simulink model "pot_field_1obs"  (R2016a)
settings: Solver=VariableStepAuto  StartTime=0.0  StopTime=inf  RelTol=1e-3
undefined symbols (not defined in the file): Speed, Yaw
libraries: robotlib x3
settings Model: Creator=nmanzini  LastModifiedBy=nmanzini

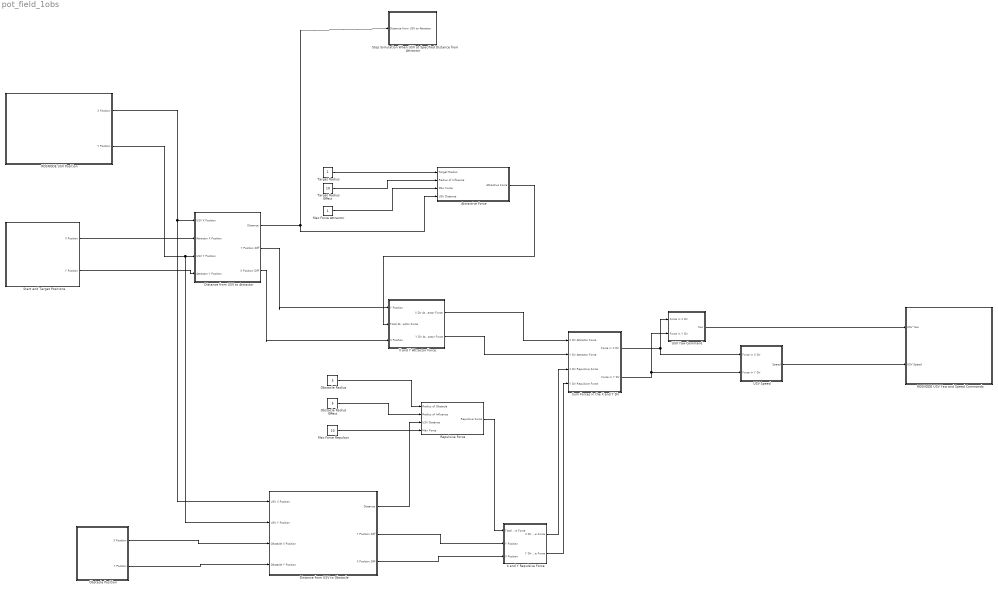
== system pot_field_1obs ==
  Attractive Force : Subsystem
  Distance from USV to Attractor : Subsystem
  Distance from USV to Obstacle : Subsystem
  Max Force Attractor : Constant  OutDataTypeStr=Inherit: Inherit via back propagation
  Max Force Repulsor : Constant  Value=10  OutDataTypeStr=Inherit: Inherit via back propagation
  "Obstacle Position " : Subsystem
  Obstacle Radius : Constant  Value=5  OutDataTypeStr=Inherit: Inherit via back propagation
  Obstacle Radius Effect : Constant  Value=5  OutDataTypeStr=Inherit: Inherit via back propagation
  ROSNODE USV Position : Subsystem
  ROSNODE USV Yaw and Speed Commands : Subsystem
  Repulsive Force : Subsystem
  Start and Target Positions : Subsystem
  Stop Simulation When USV at Specified Distance from Attractor : Subsystem
  Sum Forces in the X and Y Dir : Subsystem
  Target Radius : Constant  OutDataTypeStr=Inherit: Inherit via back propagation
  Target Radius Effect : Constant  Value=10  OutDataTypeStr=Inherit: Inherit via back propagation
  USV Speed : Subsystem
  USV Yaw Command : Subsystem
  X and Y Attractor Force : Subsystem
  X and Y Repulsive Force : Subsystem
  wires:
  Obstacle Radius/1 -> Repulsive Force/1("Radius of Obstacle ")
  Obstacle Radius Effect/1 -> Repulsive Force/2(Radius of Influence)
  Max Force Repulsor/1 -> Repulsive Force/4(Max Force)
  Repulsive Force/1(Repulsive Force) -> X and Y Repulsive Force/1(Total Repulsive Force)
  Distance from USV to Attractor/1(Distance) -> Attractive Force/4(USV Distance), Stop Simulation When USV at Specified Distance from Attractor/1(Distance from USV to Attractor)
  Start and Target Positions/1(X Position) -> Distance from USV to Attractor/2(Attractor X Position)
  Start and Target Positions/2(Y Position) -> Distance from USV to Attractor/4(Attractor Y Position)
  Distance from USV to Attractor/2(Y Position Diff) -> X and Y Attractor Force/1(Y Position)
  Distance from USV to Attractor/3(X Position Diff) -> X and Y Attractor Force/3("X Position ")
  Target Radius/1 -> Attractive Force/1(Target Radius)
  Target Radius Effect/1 -> Attractive Force/2(Radius of Influence)
  Max Force Attractor/1 -> Attractive Force/3(Max Force)
  Attractive Force/1(Attractive Force) -> X and Y Attractor Force/2(Total Attractor Force)
  Sum Forces in the X and Y Dir/1(Force in X Dir) -> USV Yaw Command/1(Force in X Dir), USV Speed/1(Force in X Dir)
  Sum Forces in the X and Y Dir/2(Force in Y Dir) -> USV Yaw Command/2("Force in Y Dir "), USV Speed/2(Force in Y Dir)
  X and Y Attractor Force/1(X Dir Attractor Force) -> Sum Forces in the X and Y Dir/1(X Dir Attractor Force)
  X and Y Attractor Force/2(Y Dir Attractor Force) -> Sum Forces in the X and Y Dir/2(Y Dir Attractor Force)
  X and Y Repulsive Force/1(X Dir Repulsive Force) -> Sum Forces in the X and Y Dir/3(X Dir Repulsive Force)
  X and Y Repulsive Force/2(Y Dir Repulsive Force) -> Sum Forces in the X and Y Dir/4("Y Dir Repulsive Force ")
  USV Yaw Command/1(Yaw) -> ROSNODE USV Yaw and Speed Commands/1(USV Yaw)
  USV Speed/1(Speed) -> ROSNODE USV Yaw and Speed Commands/2(USV Speed)
  ROSNODE USV Position/1(X Position) -> Distance from USV to Obstacle/1("USV X Position "), Distance from USV to Attractor/1(USV X Position)
  ROSNODE USV Position/2(Y Position) -> Distance from USV to Obstacle/2(USV Y Position), Distance from USV to Attractor/3(USV Y Position)
  Distance from USV to Obstacle/1(Distance) -> Repulsive Force/3(USV Distance)
  Distance from USV to Obstacle/2(Y Position Diff) -> X and Y Repulsive Force/2(Y Position)
  Distance from USV to Obstacle/3(X Position Diff) -> X and Y Repulsive Force/3(X Position)
  "Obstacle Position "/1(X Position) -> Distance from USV to Obstacle/3(Obstacle X Position)
  "Obstacle Position "/2(Y Position) -> Distance from USV to Obstacle/4(Obstacle Y Position)

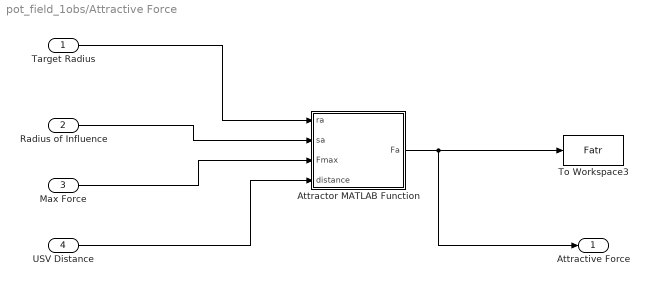
== system pot_field_1obs/Attractive Force ==
  Target Radius : Inport
  Radius of Influence : Inport  Port=2
  Max Force : Inport  Port=3
  USV Distance : Inport  Port=4
  Attractor MATLAB Function : MATLAB Function  TreatAsAtomicUnit=on
  To Workspace3 : ToWorkspace  VariableName=Fatr  SaveFormat=Timeseries  SampleTime=-1
  Attractive Force : Outport
  wires:
  Max Force/1 -> Attractor MATLAB Function/3(Fmax)
  USV Distance/1 -> Attractor MATLAB Function/4(distance)
  Attractor MATLAB Function/1(Fa) -> Attractive Force/1, To Workspace3/1
  Target Radius/1 -> Attractor MATLAB Function/1(ra)
  Radius of Influence/1 -> Attractor MATLAB Function/2(sa)

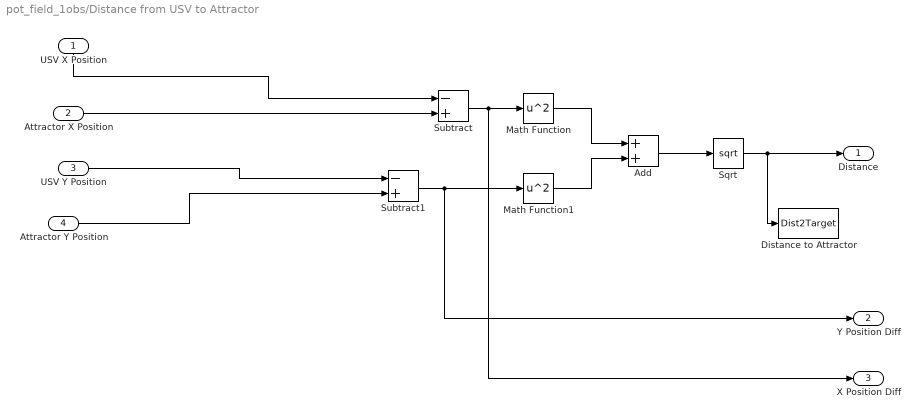
== system pot_field_1obs/Distance from USV to Attractor ==
  USV X Position : Inport
  Attractor X Position : Inport  Port=2
  USV Y Position : Inport  Port=3
  Attractor Y Position : Inport  Port=4
  Add : Sum  OutDataTypeStr=Inherit: Inherit via back propagation
  Distance to Attractor : ToWorkspace  VariableName=Dist2Target  SaveFormat=Timeseries  SampleTime=-1
  Math Function : Math  Operator=square  OutDataTypeStr=Inherit: Inherit via back propagation  SaturateOnIntegerOverflow=on
  Math Function1 : Math  Operator=square  OutDataTypeStr=Inherit: Inherit via back propagation  SaturateOnIntegerOverflow=on
  Sqrt : Sqrt  OutDataTypeStr=Inherit: Inherit via back propagation  SaturateOnIntegerOverflow=on
  Subtract : Sum  Inputs=-+  OutDataTypeStr=Inherit: Inherit via back propagation
  Subtract1 : Sum  Inputs=-+  OutDataTypeStr=Inherit: Inherit via back propagation
  Distance : Outport
  Y Position Diff : Outport  Port=2
  X Position Diff : Outport  Port=3
  wires:
  Attractor Y Position/1 -> Subtract1/2
  USV Y Position/1 -> Subtract1/1
  USV X Position/1 -> Subtract/1
  Attractor X Position/1 -> Subtract/2
  Subtract1/1 -> Y Position Diff/1, Math Function1/1
  Subtract/1 -> X Position Diff/1, Math Function/1
  Math Function/1 -> Add/1
  Math Function1/1 -> Add/2
  Add/1 -> Sqrt/1
  Sqrt/1 -> Distance/1, Distance to Attractor/1

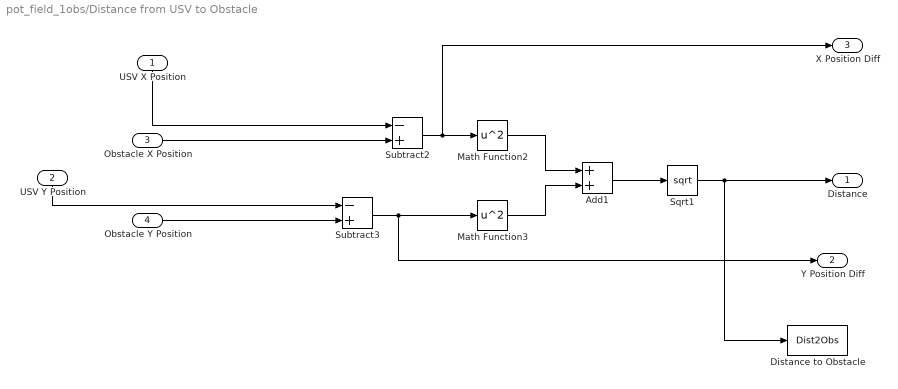
== system pot_field_1obs/Distance from USV to Obstacle ==
  "USV X Position " : Inport
  USV Y Position : Inport  Port=2
  Obstacle X Position : Inport  Port=3
  Obstacle Y Position : Inport  Port=4
  Add1 : Sum  OutDataTypeStr=Inherit: Inherit via back propagation
  Distance to Obstacle : ToWorkspace  VariableName=Dist2Obs  SaveFormat=Timeseries  SampleTime=-1
  Math Function2 : Math  Operator=square  OutDataTypeStr=Inherit: Inherit via back propagation  SaturateOnIntegerOverflow=on
  Math Function3 : Math  Operator=square  OutDataTypeStr=Inherit: Inherit via back propagation  SaturateOnIntegerOverflow=on
  Sqrt1 : Sqrt  OutDataTypeStr=Inherit: Inherit via back propagation  SaturateOnIntegerOverflow=on
  Subtract2 : Sum  Inputs=-+  OutDataTypeStr=Inherit: Inherit via back propagation
  Subtract3 : Sum  Inputs=-+  OutDataTypeStr=Inherit: Inherit via back propagation
  Distance : Outport
  Y Position Diff : Outport  Port=2
  X Position Diff : Outport  Port=3
  wires:
  Sqrt1/1 -> Distance/1, Distance to Obstacle/1
  Subtract3/1 -> Y Position Diff/1, Math Function3/1
  Subtract2/1 -> X Position Diff/1, Math Function2/1
  Obstacle X Position/1 -> Subtract2/2
  "USV X Position "/1 -> Subtract2/1
  Obstacle Y Position/1 -> Subtract3/2
  USV Y Position/1 -> Subtract3/1
  Math Function2/1 -> Add1/1
  Math Function3/1 -> Add1/2
  Add1/1 -> Sqrt1/1

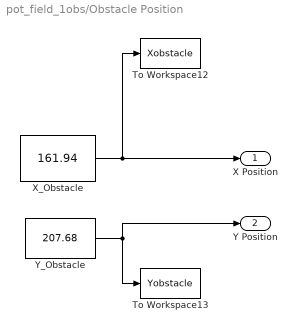
== system pot_field_1obs/Obstacle Position  ==
  To Workspace12 : ToWorkspace  VariableName=Xobstacle  SaveFormat=Timeseries  SampleTime=-1
  To Workspace13 : ToWorkspace  VariableName=Yobstacle  SaveFormat=Timeseries  SampleTime=-1
  "X_Obstacle " : Constant  Value=161.94  OutDataTypeStr=Inherit: Inherit via back propagation
  Y_Obstacle : Constant  Value=207.68  OutDataTypeStr=Inherit: Inherit via back propagation
  X Position : Outport
  Y Position : Outport  Port=2
  wires:
  "X_Obstacle "/1 -> X Position/1, To Workspace12/1
  Y_Obstacle/1 -> Y Position/1, To Workspace13/1

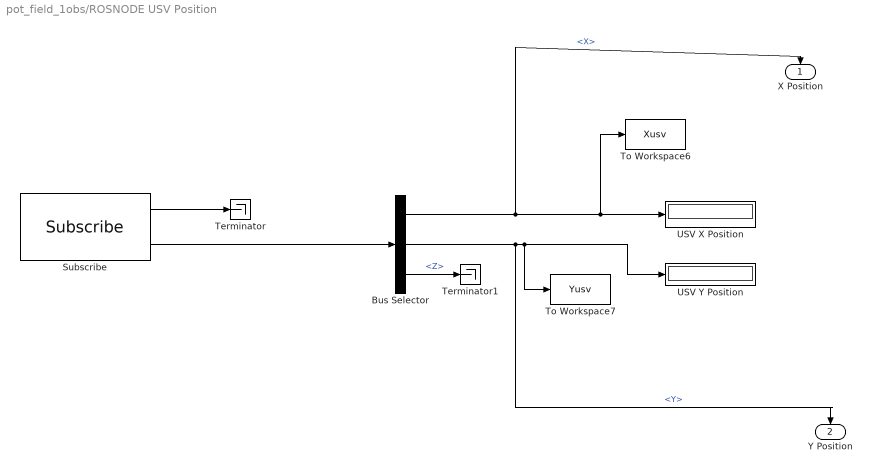
== system pot_field_1obs/ROSNODE USV Position ==
  Bus Selector : BusSelector  OutputSignals=Pose.Pose.Position.X,Pose.Pose.Position.Y,Pose.Pose.Position.Z
  Subscribe : robotlib/Subscribe  SourceLibraryInfo=This block requires Robotics System Toolbox  topicSource=Select from ROS network  topic=/geonav_odom  messageType=nav_msgs/Odometry  sampleTime=-1  messageQueueLength=1000
  Terminator : Terminator
  Terminator1 : Terminator
  To Workspace6 : ToWorkspace  VariableName=Xusv  SaveFormat=Timeseries  SampleTime=-1
  To Workspace7 : ToWorkspace  VariableName=Yusv  SaveFormat=Timeseries  SampleTime=-1
  USV X Position : Display
  USV Y Position : Display
  X Position : Outport
  Y Position : Outport  Port=2
  wires:
  Subscribe/1 -> Terminator/1
  Bus Selector/3 -> Terminator1/1  "<Z>"
  Bus Selector/1 -> X Position/1, To Workspace6/1, USV X Position/1  "<X>"
  Subscribe/2 -> Bus Selector/1
  Bus Selector/2 -> USV Y Position/1, To Workspace7/1, Y Position/1  "<Y>"

== system pot_field_1obs/ROSNODE USV Yaw and Speed Commands ==
  USV Yaw : Inport
  USV Speed : Inport  Port=2
  Blank Message : robotlib/Blank Message  SourceLibraryInfo=This block requires Robotics System Toolbox  messageType=kingfisher_msgs/Course  SampleTime=inf
  Bus Assignment : BusAssignment  AssignedSignals=Yaw,Speed
  Publish1 : robotlib/Publish  SourceLibraryInfo=This block requires Robotics System Toolbox  topicSource=Select from ROS network  topic=/cmd_course  messageType=kingfisher_msgs/Course  messageQueueLength=1
  wires:
  USV Speed/1 -> Bus Assignment/3
  USV Yaw/1 -> Bus Assignment/2
  Blank Message/1 -> Bus Assignment/1
  Bus Assignment/1 -> Publish1/1

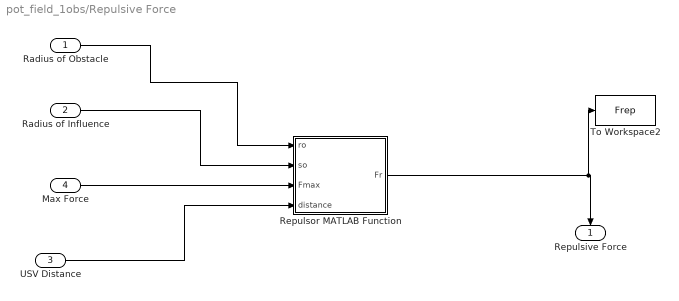
== system pot_field_1obs/Repulsive Force ==
  "Radius of Obstacle " : Inport
  Radius of Influence : Inport  Port=2
  USV Distance : Inport  Port=3
  Max Force : Inport  Port=4
  Repulsor MATLAB Function : MATLAB Function  TreatAsAtomicUnit=on
  To Workspace2 : ToWorkspace  VariableName=Frep  SaveFormat=Timeseries  SampleTime=-1
  Repulsive Force : Outport
  wires:
  USV Distance/1 -> Repulsor MATLAB Function/4(distance)
  Repulsor MATLAB Function/1(Fr) -> Repulsive Force/1, To Workspace2/1
  Max Force/1 -> Repulsor MATLAB Function/3(Fmax)
  Radius of Influence/1 -> Repulsor MATLAB Function/2(so)
  "Radius of Obstacle "/1 -> Repulsor MATLAB Function/1(ro)

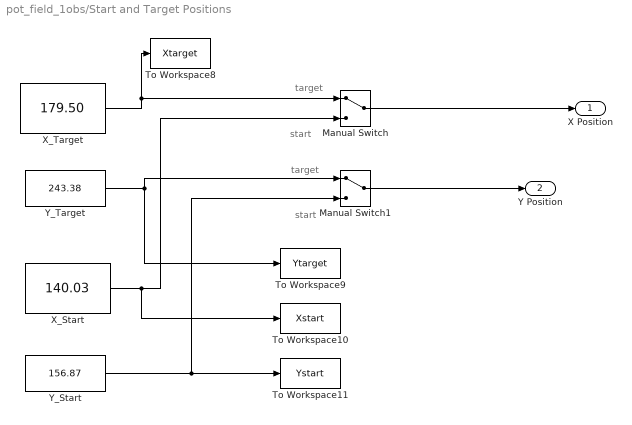
== system pot_field_1obs/Start and Target Positions ==
  note: target
  note: target
  note: start
  note: start
  Manual Switch : ManualSwitch
  Manual Switch1 : ManualSwitch
  To Workspace10 : ToWorkspace  VariableName=Xstart  SaveFormat=Timeseries  SampleTime=-1
  To Workspace11 : ToWorkspace  VariableName=Ystart  SaveFormat=Timeseries  SampleTime=-1
  To Workspace8 : ToWorkspace  VariableName=Xtarget  SaveFormat=Timeseries  SampleTime=-1
  To Workspace9 : ToWorkspace  VariableName=Ytarget  SaveFormat=Timeseries  SampleTime=-1
  X_Start : Constant  Value=140.03  OutDataTypeStr=Inherit: Inherit via back propagation
  X_Target : Constant  Value=179.50  OutDataTypeStr=Inherit: Inherit via back propagation
  Y_Start : Constant  Value=156.87  OutDataTypeStr=Inherit: Inherit via back propagation
  Y_Target : Constant  Value=243.38  OutDataTypeStr=Inherit: Inherit via back propagation
  X Position : Outport
  Y Position : Outport  Port=2
  wires:
  X_Target/1 -> To Workspace8/1, Manual Switch/1
  Manual Switch/1 -> X Position/1
  X_Start/1 -> To Workspace10/1, Manual Switch/2
  Y_Target/1 -> To Workspace9/1, Manual Switch1/1
  Manual Switch1/1 -> Y Position/1
  Y_Start/1 -> To Workspace11/1, Manual Switch1/2

== system pot_field_1obs/Stop Simulation When USV at Specified Distance from Attractor ==
  Distance from USV to Attractor : Inport
  Display1 : Display
  Stop Gain1 : Constant  Value=0  OutDataTypeStr=Inherit: Inherit via back propagation
  Stop Gain2 : Constant  OutDataTypeStr=Inherit: Inherit via back propagation
  Stop Simulation : Stop
  Stop Simulation Switch at distance from Target : Switch  Criteria=u2 > Threshold  Threshold=1.5
  wires:
  Distance from USV to Attractor/1 -> Stop Simulation Switch at distance from Target/2
  Stop Simulation Switch at distance from Target/1 -> Display1/1, Stop Simulation/1
  Stop Gain1/1 -> Stop Simulation Switch at distance from Target/1
  Stop Gain2/1 -> Stop Simulation Switch at distance from Target/3

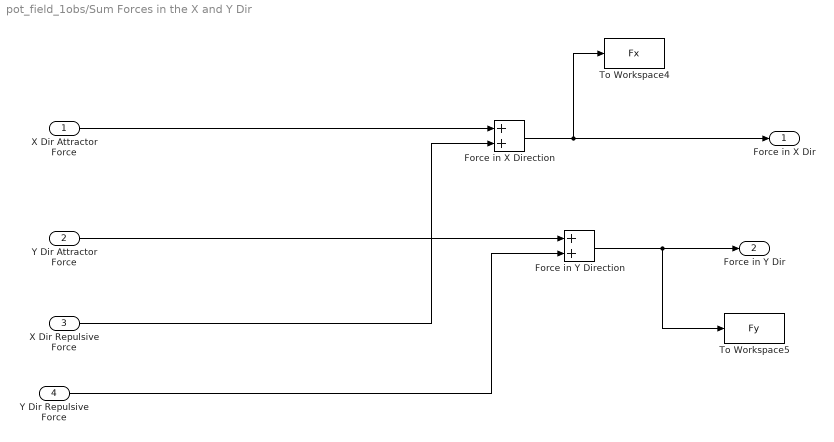
== system pot_field_1obs/Sum Forces in the X and Y Dir ==
  X Dir Attractor Force : Inport
  Y Dir Attractor Force : Inport  Port=2
  X Dir Repulsive Force : Inport  Port=3
  "Y Dir Repulsive Force " : Inport  Port=4
  Force in X Direction : Sum  OutDataTypeStr=Inherit: Inherit via back propagation
  Force in Y Direction : Sum  OutDataTypeStr=Inherit: Inherit via back propagation
  To Workspace4 : ToWorkspace  VariableName=Fx  SaveFormat=Timeseries  SampleTime=-1
  To Workspace5 : ToWorkspace  VariableName=Fy  SaveFormat=Timeseries  SampleTime=-1
  Force in X Dir : Outport
  Force in Y Dir : Outport  Port=2
  wires:
  X Dir Attractor Force/1 -> Force in X Direction/1
  X Dir Repulsive Force/1 -> Force in X Direction/2
  "Y Dir Repulsive Force "/1 -> Force in Y Direction/2
  Y Dir Attractor Force/1 -> Force in Y Direction/1
  Force in Y Direction/1 -> Force in Y Dir/1, To Workspace5/1
  Force in X Direction/1 -> Force in X Dir/1, To Workspace4/1

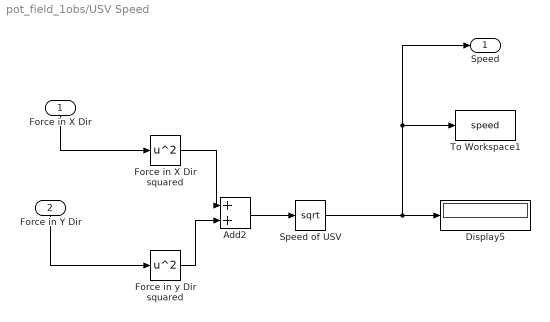
== system pot_field_1obs/USV Speed ==
  Force in X Dir : Inport
  Force in Y Dir : Inport  Port=2
  Add2 : Sum  OutDataTypeStr=Inherit: Inherit via back propagation
  Display5 : Display
  Force in X Dir squared : Math  Operator=square  OutDataTypeStr=Inherit: Inherit via back propagation  SaturateOnIntegerOverflow=on
  Force in y Dir squared : Math  Operator=square  OutDataTypeStr=Inherit: Inherit via back propagation  SaturateOnIntegerOverflow=on
  Speed of USV : Sqrt  OutDataTypeStr=Inherit: Inherit via back propagation  SaturateOnIntegerOverflow=on
  To Workspace1 : ToWorkspace  VariableName=speed  SaveFormat=Timeseries  SampleTime=-1
  Speed : Outport
  wires:
  Force in X Dir/1 -> Force in X Dir squared/1
  Force in Y Dir/1 -> Force in y Dir squared/1
  Speed of USV/1 -> Speed/1, To Workspace1/1, Display5/1
  Force in X Dir squared/1 -> Add2/1
  Force in y Dir squared/1 -> Add2/2
  Add2/1 -> Speed of USV/1

== system pot_field_1obs/USV Yaw Command ==
  Force in X Dir : Inport
  "Force in Y Dir " : Inport  Port=2
  Display2 : Display
  Heading of the USV : Trigonometry  Operator=atan2
  To Workspace : ToWorkspace  VariableName=yaw  SaveFormat=Timeseries  SampleTime=-1
  Yaw : Outport
  wires:
  "Force in Y Dir "/1 -> Heading of the USV/1
  Force in X Dir/1 -> Heading of the USV/2
  Heading of the USV/1 -> Display2/1, Yaw/1, To Workspace/1

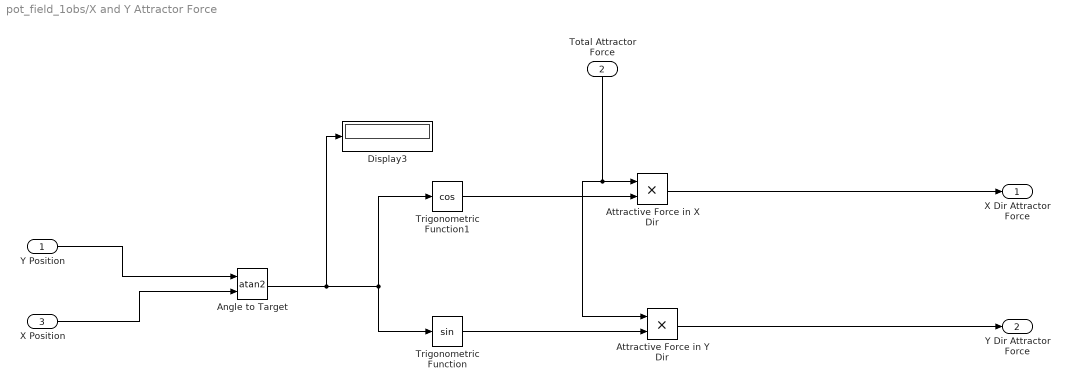
== system pot_field_1obs/X and Y Attractor Force ==
  Y Position : Inport
  Total Attractor Force : Inport  Port=2
  "X Position " : Inport  Port=3
  Angle to Target : Trigonometry  Operator=atan2
  Attractive Force in X Dir : Product  OutDataTypeStr=Inherit: Inherit via back propagation
  Attractive Force in Y Dir : Product  OutDataTypeStr=Inherit: Inherit via back propagation
  Display3 : Display
  Trigonometric Function : Trigonometry
  Trigonometric Function1 : Trigonometry  Operator=cos
  X Dir Attractor Force : Outport
  Y Dir Attractor Force : Outport  Port=2
  wires:
  Y Position/1 -> Angle to Target/1
  "X Position "/1 -> Angle to Target/2
  Angle to Target/1 -> Display3/1, Trigonometric Function1/1, Trigonometric Function/1
  Trigonometric Function1/1 -> Attractive Force in X Dir/2
  Trigonometric Function/1 -> Attractive Force in Y Dir/2
  Attractive Force in X Dir/1 -> X Dir Attractor Force/1
  Attractive Force in Y Dir/1 -> Y Dir Attractor Force/1
  Total Attractor Force/1 -> Attractive Force in Y Dir/1, Attractive Force in X Dir/1

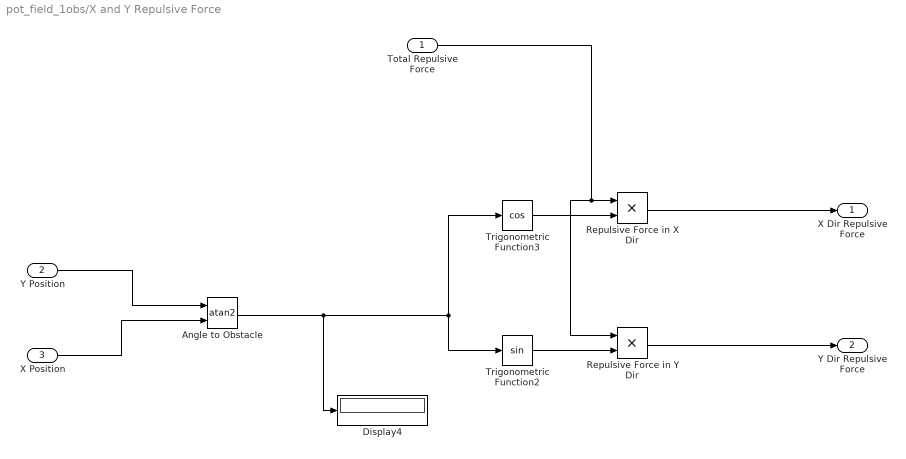
== system pot_field_1obs/X and Y Repulsive Force ==
  Total Repulsive Force : Inport
  Y Position : Inport  Port=2
  X Position : Inport  Port=3
  Angle to Obstacle : Trigonometry  Operator=atan2
  Display4 : Display
  Repulsive Force in X Dir : Product  OutDataTypeStr=Inherit: Inherit via back propagation
  Repulsive Force in Y Dir : Product  OutDataTypeStr=Inherit: Inherit via back propagation
  Trigonometric Function2 : Trigonometry
  Trigonometric Function3 : Trigonometry  Operator=cos
  X Dir Repulsive Force : Outport
  Y Dir Repulsive Force : Outport  Port=2
  wires:
  X Position/1 -> Angle to Obstacle/2
  Y Position/1 -> Angle to Obstacle/1
  Total Repulsive Force/1 -> Repulsive Force in Y Dir/1, Repulsive Force in X Dir/1
  Angle to Obstacle/1 -> Display4/1, Trigonometric Function3/1, Trigonometric Function2/1
  Trigonometric Function2/1 -> Repulsive Force in Y Dir/2
  Repulsive Force in X Dir/1 -> X Dir Repulsive Force/1
  Repulsive Force in Y Dir/1 -> Y Dir Repulsive Force/1
  Trigonometric Function3/1 -> Repulsive Force in X Dir/2

== matlab function pot_field_1obs/Repulsive Force/Repulsor MATLAB Function ==
  data: ro input; Fr output; so input; Fmax input; distance input
function Fr = fcn(ro, so, Fmax, distance)
%#codegen

%Repulsor if statement
%distance - distance from USV to obstacle
%ro - radius of obstacle in meters
%so - radius of influence of obstacle in meters
%Fr - replusive force in newtons
%Fmax - max force in newtons

if distance < ro
    
    Fr = -1*Fmax;
    
elseif distance <= (so + ro)
    
    Fr = -1*Fmax*(1 - ((distance - ro)/so));
    
else
    
    Fr = 0;
    
end
    
end

== matlab function pot_field_1obs/Attractive Force/Attractor MATLAB Function ==
  data: ra input; Fa output; sa input; Fmax input; distance input
function Fa = fcn(ra, sa, Fmax, distance)
%#codegen

%Attractor if statement
%distance - distance from USV to attractor
%ra - radius of attractor in meters
%sa - radius of influence in meters
%Fa - attractor force in newtons
%Fmax - max force in newtons

if distance < ra
    
    Fa = 0;
    
elseif distance <= (sa + ra)
    
    Fa = Fmax *((distance - ra)/sa);
    
else
    
    Fa = Fmax;
    
end
    
end
